simulink subsystem "StateMachine"  (R2024a)
settings: Solver=VariableStepAuto  StartTime=0.0  StopTime=10.0  RelTol=1e-3
undefined symbols (not defined in the file or in its folder): system_enable
settings Model: Creator=20192648  LastModifiedBy=20192648

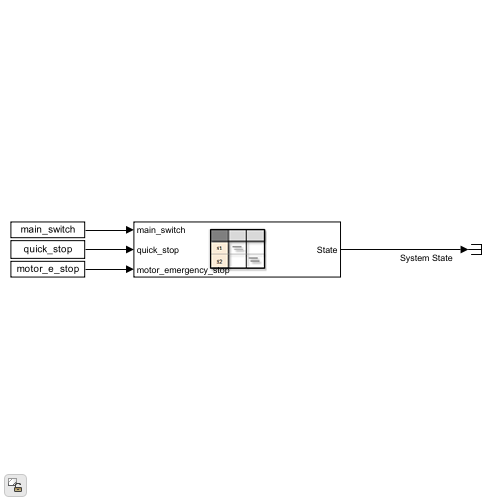
[thumbnail: Simulink's stored preview of the top-level diagram]
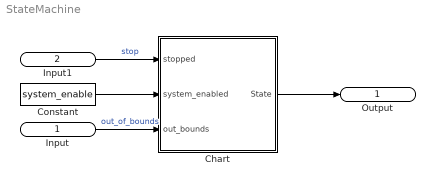
== system StateMachine ==
  Input : Inport
  Input1 : Inport  Port=2
  Chart : Stateflow chart  TreatAsAtomicUnit=on
  Constant : Constant  Value=system_enable  OutDataTypeStr=boolean
  Output : Outport
  wires:
  Chart/1(State) -> Output/1
  Input/1 -> Chart/3(out_bounds)  "out_of_bounds"
  Input1/1 -> Chart/1(stopped)  "stop"
  Constant/1 -> Chart/2(system_enabled)

== stateflow chart StateMachine/Chart ==
  settings: sampleTime=0.01  executeAtInitialization=1
  state Not_Stopped
    state Idle
    state Running
    state Out_of_Bounds
    (default) -> Idle
    Not_Stopped -> Idle [order 1] : [~system_enabled]
    Idle -> Running : [system_enabled]
    Out_of_Bounds -> Running : [~out_bounds]
    Running -> Out_of_Bounds : [out_bounds]
  state Stopped
  (default) -> Not_Stopped
  Stopped -> Not_Stopped : [~system_enabled]
  Not_Stopped -> Stopped [order 1] : [stopped]
  data: stopped input; State output Enum: SystemStateEnum; system_enabled input; out_bounds input
